simulink model "vehicle_ev"  (R2017a)
settings: Solver=FixedStepDiscrete  StartTime=0.0  StopTime=inf  FixedStep=abs(Ts)  RelTol=1e-3
InitFcn:
  | if ~exist('Ts')
  |     Ts = 1;
  | end
undefined symbols (not defined in the file or in its folder): elvio_cycle_wltp_3b
libraries: elvio x9
settings Model: Creator=tstef  LastModifiedBy=tstef

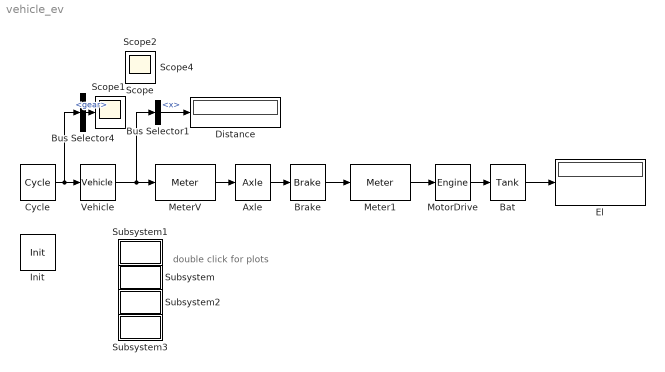
== system vehicle_ev ==
  note: double click
      | for plots
  Axle : elvio/Drive/Axle  radius=0.3  ratio=4  factor=0.1  FromTag1=Axle1  GotoTag1=MeterV1
  Bat : elvio/Drive/Tank  GotoTag1=MotorDrive1
  Brake : elvio/Drive/Brake  Tbrake=5000  FromTag1=Brake1  GotoTag1=Axle1
  Bus Selector1 : BusSelector  OutputSignals=info.x
  Bus Selector4 : BusSelector  OutputSignals=gear
  Cycle : elvio/Drive/Cycle  data=elvio_cycle_wltp_3b()  acc=-3
  Distance : Display
  El : Display
  Init : elvio/Drive/Init  Ts0=1
  Meter1 : elvio/Drive/Meter  d=100  FromTag1=Meter11  GotoTag1=Brake1
  MeterV : elvio/Drive/Meter  d=100  FromTag1=MeterV1  GotoTag1=Vehicle1
  MotorDrive : elvio/Drive/Engine  Tmax=60  Tmin=-60  Tfrict=0.2  Ploss=100  lossf=0.01  lossnorm=2e6  lossR=0.05  FromTag1=MotorDrive1  GotoTag1=Meter11
  Scope{,1..2,4} (4 alike) : Scope
      Scope4 mask Display: disp('1.484e+07')
  Subsystem : Subsystem
      settings: OpenFcn=elvio_plot_scatter(logsout);
      mask Display: disp('Scatter')
  Subsystem1 : Subsystem
      settings: OpenFcn=elvio_plot_energy(logsout);
      mask Display: disp('Energy')
  Subsystem2 : Subsystem
      settings: OpenFcn=elvio_plot_sources(logsout);
      mask Display: disp('Sources')
  Subsystem3 : Subsystem
      settings: OpenFcn=elvio_plot_sources_xy(logsout);
      mask Display: disp('Srcs. xy')
  Vehicle : elvio/Drive/Vehicle  m=1200  Froll=150  Aeff=0.3  n=[1 5]  FromTag1=Vehicle1
  wires:
  Vehicle/1 -> MeterV/1, Bus Selector1/1
  MotorDrive/1 -> Bat/1
  Bat/1 -> El/1
  Bus Selector1/1 -> Distance/1  "<x>"
  Meter1/1 -> MotorDrive/1
  MeterV/1 -> Axle/1
  Cycle/1 -> Bus Selector4/1, Vehicle/1
  Bus Selector4/1 -> Scope1/1  "<gear>"
  Axle/1 -> Brake/1
  Brake/1 -> Meter1/1

== system vehicle_ev/Subsystem ==

== system vehicle_ev/Subsystem1 ==

== system vehicle_ev/Subsystem2 ==

== system vehicle_ev/Subsystem3 ==
